simulink model "lechape_ex2_simu"  (R2023a)
settings: Solver=VariableStepAuto  StartTime=0.0  StopTime=Tsim  RelTol=1e-3
values from neighbouring files (symbols this model uses):
  A = [0 1; -9 3]    [lechape_ex1_code.m]    (also in lechape_ex2_code.m)
  B = [0 1]'    [lechape_ex1_code.m]    (also in lechape_ex2_code.m)
  h = 0.5    [lechape_ex1_code.m]    (also in lechape_ex2_code.m)
  K = [-45 -18]    [lechape_ex2_code.m]
  N = 500    [lechape_ex1_code.m]    (also in lechape_ex2_code.m)
  x0 = [1.5; 1]    [lechape_ex2_code.m]
undefined symbols (not defined in the file or in its folder): Ad, Bd, Cd, Dd, KSoma, Q, tal
settings Model: Creator=Vasco  LastModifiedBy=Vasco
settings DataIOCC: ReturnWorkspaceOutputs=off

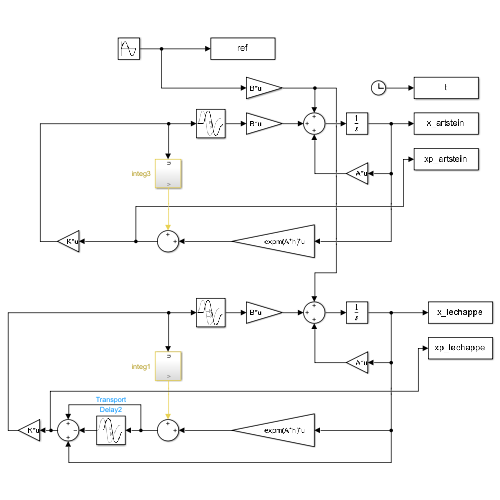
[thumbnail: Simulink's stored preview of the top-level diagram]
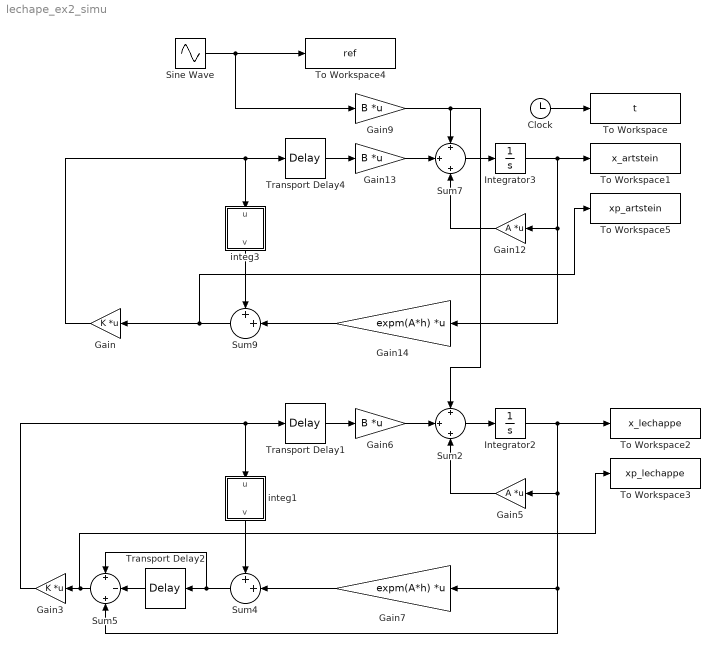
== system lechape_ex2_simu ==
  Clock : Clock
  Gain : Gain  Gain=K  Multiplication=Matrix(K*u)
  Gain12 : Gain  Gain=A  Multiplication=Matrix(K*u)
  Gain13 : Gain  Gain=B  Multiplication=Matrix(K*u)
  Gain14 : Gain  Gain=expm(A*h)  Multiplication=Matrix(K*u)
  Gain3 : Gain  Gain=K  Multiplication=Matrix(K*u)
  Gain5 : Gain  Gain=A  Multiplication=Matrix(K*u)
  Gain6 : Gain  Gain=B  Multiplication=Matrix(K*u)
  Gain7 : Gain  Gain=expm(A*h)  Multiplication=Matrix(K*u)
  Gain9 : Gain  Gain=B  Multiplication=Matrix(K*u)
  Integrator2 : Integrator  InitialCondition=x0
  Integrator3 : Integrator  InitialCondition=x0
  Sine Wave : Sin  Amplitude=3  Frequency=0.5  SampleTime=0
  Sum2 : Sum  Inputs=+|+|+
  Sum4 : Sum  Inputs=++|
  Sum5 : Sum  Inputs=+|-|+
  Sum7 : Sum  Inputs=+|+|+
  Sum9 : Sum  Inputs=++|
  To Workspace : ToWorkspace  VariableName=t  SampleTime=-1
  To Workspace1 : ToWorkspace  VariableName=x_artstein  SampleTime=-1
  To Workspace2 : ToWorkspace  VariableName=x_lechappe  SampleTime=-1
  To Workspace3 : ToWorkspace  VariableName=xp_lechappe  SampleTime=-1
  To Workspace4 : ToWorkspace  VariableName=ref  SampleTime=-1
  To Workspace5 : ToWorkspace  VariableName=xp_artstein  SampleTime=-1
  Transport Delay1 : TransportDelay  DelayTime=h
  Transport Delay2 : TransportDelay  DelayTime=h
  Transport Delay4 : TransportDelay  DelayTime=h
  integ1 : Subsystem
  integ3 : Subsystem
  wires:
  Clock/1 -> To Workspace/1
  integ3/1(v) -> Sum9/1
  Gain13/1 -> Sum7/2
  Gain12/1 -> Sum7/3
  Sum7/1 -> Integrator3/1
  Transport Delay4/1 -> Gain13/1
  Gain14/1 -> Sum9/2
  Integrator3/1 -> Gain14/1, Gain12/1, To Workspace1/1
  Gain5/1 -> Sum2/3
  integ1/1(v) -> Sum4/1
  Sum2/1 -> Integrator2/1
  Gain7/1 -> Sum4/2
  Gain6/1 -> Sum2/2
  Transport Delay1/1 -> Gain6/1
  Sum5/1 -> Gain3/1, To Workspace3/1
  Sum4/1 -> Transport Delay2/1, Sum5/1
  Transport Delay2/1 -> Sum5/2
  Gain9/1 -> Sum7/1, Sum2/1
  Sine Wave/1 -> Gain9/1, To Workspace4/1
  Sum9/1 -> Gain/1, To Workspace5/1
  Gain3/1 -> integ1/1(u), Transport Delay1/1
  Gain/1 -> Transport Delay4/1, integ3/1(u)
  Integrator2/1 -> Sum5/3, Gain7/1, Gain5/1, To Workspace2/1

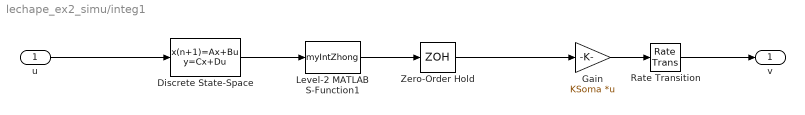
== system lechape_ex2_simu/integ1 ==
  u : Inport
  Discrete State-Space : DiscreteStateSpace  A=Ad  B=Bd  C=Cd  D=Dd  SampleTime=tal
  Gain : Gain  Gain=KSoma  Multiplication=Matrix(K*u)
  Level-2 MATLAB S-Function1 : M-S-Function  FunctionName=myIntZhong  Parameters=tal,A,B,Q,N
  Rate Transition : RateTransition
  Zero-Order Hold : ZeroOrderHold  SampleTime=tal
  v : Outport  VectorParamsAs1DForOutWhenUnconnected=off
  wires:
  Rate Transition/1 -> v/1
  u/1 -> Discrete State-Space/1
  Gain/1 -> Rate Transition/1
  Zero-Order Hold/1 -> Gain/1
  Discrete State-Space/1 -> Level-2 MATLAB S-Function1/1
  Level-2 MATLAB S-Function1/1 -> Zero-Order Hold/1

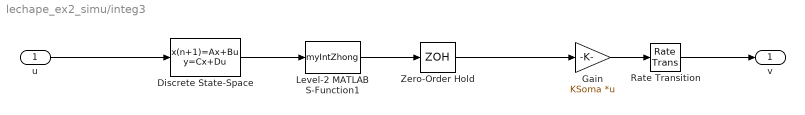
== system lechape_ex2_simu/integ3 ==
  u : Inport
  Discrete State-Space : DiscreteStateSpace  A=Ad  B=Bd  C=Cd  D=Dd  SampleTime=tal
  Gain : Gain  Gain=KSoma  Multiplication=Matrix(K*u)
  Level-2 MATLAB S-Function1 : M-S-Function  FunctionName=myIntZhong  Parameters=tal,A,B,Q,N
  Rate Transition : RateTransition
  Zero-Order Hold : ZeroOrderHold  SampleTime=tal
  v : Outport  VectorParamsAs1DForOutWhenUnconnected=off
  wires:
  Rate Transition/1 -> v/1
  u/1 -> Discrete State-Space/1
  Gain/1 -> Rate Transition/1
  Zero-Order Hold/1 -> Gain/1
  Discrete State-Space/1 -> Level-2 MATLAB S-Function1/1
  Level-2 MATLAB S-Function1/1 -> Zero-Order Hold/1
